simulink model "scdmrate_ol"  (Simulink 7.6)
settings: Solver=ode45  StartTime=0.0  StopTime=100  RelTol=1e-3
model workspace (MAT data in the model file):
  sysC = zpk
  sysC.IOSize_ = [1 1]
  sysC.Data_ = ltipack.zpkdata
  sysC.Data_.z = {-2}
  sysC.Data_.p = {-10}
  sysC.Data_.k = 0.1
  sysC.Data_.Delay.Input = 0
  sysC.Data_.Delay.Output = 0
  sysC.Data_.Delay.IO = 0
  sysC.Data_.Ts = 0
  sysC.Data_.Tags = struct()
  sysTs1 = zpk
  sysTs1.IOSize_ = [1 1]
  sysTs1.Data_ = ltipack.zpkdata
  sysTs1.Data_.z = {-0.7463}
  sysTs1.Data_.p = {[0.4251; 0.9735]}
  sysTs1.Data_.k = 0.2212
  sysTs1.Data_.Delay.Input = 0
  sysTs1.Data_.Delay.Output = 0
  sysTs1.Data_.Delay.IO = 0
  sysTs1.Data_.Ts = 0.01
  sysTs1.Data_.Tags = struct()
  sysTs2 = zpk
  sysTs2.IOSize_ = [1 1]
  sysTs2.Data_ = ltipack.zpkdata
  sysTs2.Data_.z = {[]}
  sysTs2.Data_.p = {0.7788}
  sysTs2.Data_.k = 0.2212
  sysTs2.Data_.Delay.Input = 0
  sysTs2.Data_.Delay.Output = 0
  sysTs2.Data_.Delay.IO = 0
  sysTs2.Data_.Ts = 0.025
  sysTs2.Data_.Tags = struct()
libraries: cstblocks x1
settings Model: Creator=The MathWorks Inc.
settings OptimizationCC: InlineInvariantSignals=on  InitFltsAndDblsToZero=on
settings DebuggingCC: SaveWithParameterizedLinksMsg=none  SignalResolutionControl=TryResolveAllWithWarning  MultiTaskDSMMsg=warning  BusObjectLabelMismatch=none  StrictBusMsg=None
settings GRTTargetCC: TargetFcnLib=ansi_tfl_tmw.mat

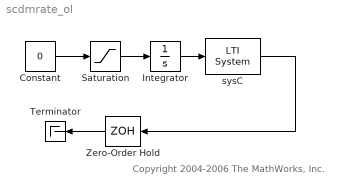
== system scdmrate_ol ==
  note: Copyright 2004-2006
      | The MathWorks, Inc.
  Constant : Constant  Value=0  SampleTime=0.01
  Integrator : Integrator
  Saturation : Saturate  UpperLimit=200  LowerLimit=200
  Terminator : Terminator
  Zero-Order Hold : ZeroOrderHold  SampleTime=0.01
  sysC : cstblocks/LTI System  SystemSampleTime=-1  sys=sysC  IC=[]
  wires:
  Constant/1 -> Saturation/1
  sysC/1 -> Zero-Order Hold/1
  Saturation/1 -> Integrator/1
  Integrator/1 -> sysC/1
  Zero-Order Hold/1 -> Terminator/1
